simulink model "overhead_crane_linearization_model"  (R2023b)
settings: Solver=VariableStepAuto  StartTime=0.0  StopTime=15  RelTol=1e-3
values from neighbouring files (symbols this model uses):
  A = modello_linearizzazione_Timed_Based_Linearization.a    [linearization_simulink_initialization.m]    (also in overhead_crane_control_initialization.m = overhead_crane_linearization_model_Timed_Based_Linearization)
  alpha_0_eq = pi/2    (= 1.57079632679)    [linearization_simulink_initialization.m]
  alpha_dot_0_eq = 0    [linearization_simulink_initialization.m]
  B = modello_linearizzazione_Timed_Based_Linearization.b    [linearization_simulink_initialization.m]    (also in overhead_crane_control_initialization.m = overhead_crane_linearization_model_Timed_Based_Linearization)
  C = modello_linearizzazione_Timed_Based_Linearization.c    [linearization_simulink_initialization.m]    (also in overhead_crane_control_initialization.m = overhead_crane_linearization_model_Timed_Based_Linearization)
  cc = 5e3    (= 5000)    [linearization_simulink_initialization.m]    (also in overhead_crane_control_initialization.m)
  cm = 100    [linearization_simulink_initialization.m]    (also in overhead_crane_control_initialization.m)
  D = modello_linearizzazione_Timed_Based_Linearization.d    [linearization_simulink_initialization.m]    (also in overhead_crane_control_initialization.m = overhead_crane_linearization_model_Timed_Based_Linearization)
  g = 9.81    [linearization_simulink_initialization.m]    (also in overhead_crane_control_initialization.m)
  L = 2.5    [linearization_simulink_initialization.m]    (also in overhead_crane_control_initialization.m)
  mc = 300    [linearization_simulink_initialization.m]    (also in overhead_crane_control_initialization.m)
  mm = 1000    [linearization_simulink_initialization.m]    (also in overhead_crane_control_initialization.m)
  xc_0_eq = 0    [linearization_simulink_initialization.m]
  xc_dot_0_eq = 0    [linearization_simulink_initialization.m]
undefined symbols (not defined in the file or in its folder): dinamica_alpha
settings Model: Creator=fabio  LastModifiedBy=lorez
settings OptimizationCC: BlockReduction=off  DefaultParameterBehavior=Inlined  BufferReuse=off  ReuseModelBlockBuffer=off

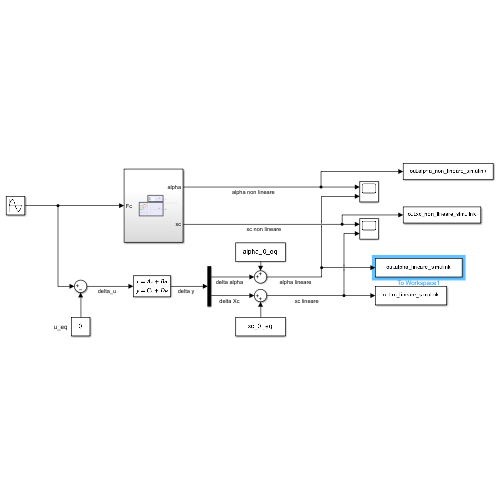
[thumbnail: Simulink's stored preview of the top-level diagram]
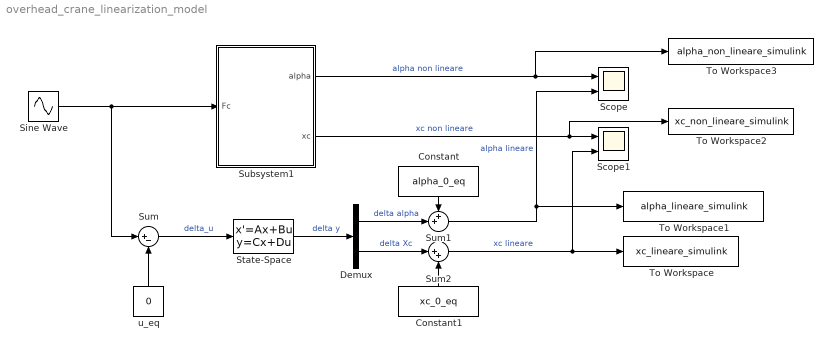
== system overhead_crane_linearization_model ==
  Constant : Constant  Value=alpha_0_eq
  Constant1 : Constant  Value=xc_0_eq
  Demux : Demux  Outputs=2
  Scope : Scope  NumInputPorts=2
  Scope1 : Scope  NumInputPorts=2
  Sine Wave : Sin  Amplitude=1e4  Frequency=2  SampleTime=0
  State-Space : StateSpace  A=A  B=B  C=C  D=D  InitialCondition=0
  Subsystem1 : Subsystem
  Sum : Sum  Inputs=|+-
  Sum1 : Sum  Inputs=++|
  Sum2 : Sum  Inputs=|++
  To Workspace : ToWorkspace  VariableName=xc_lineare_simulink  SampleTime=-1
  To Workspace1 : ToWorkspace  VariableName=alpha_lineare_simulink  SampleTime=-1
  To Workspace2 : ToWorkspace  VariableName=xc_non_lineare_simulink  SampleTime=-1
  To Workspace3 : ToWorkspace  VariableName=alpha_non_lineare_simulink  SampleTime=-1
  u_eq : Constant  Value=0
  wires:
  Subsystem1/1(alpha) -> To Workspace3/1, Scope/1  "alpha non lineare"
  Subsystem1/2(xc) -> To Workspace2/1, Scope1/1  "xc non lineare"
  Sine Wave/1 -> Sum/1, Subsystem1/1(Fc)
  Sum/1 -> State-Space/1  "delta_u"
  u_eq/1 -> Sum/2
  State-Space/1 -> Demux/1  "delta y"
  Demux/1 -> Sum1/2  "delta alpha"
  Constant/1 -> Sum1/1
  Demux/2 -> Sum2/1  "delta Xc"
  Constant1/1 -> Sum2/2
  Sum1/1 -> Scope/2, To Workspace1/1  "alpha lineare"
  Sum2/1 -> Scope1/2, To Workspace/1  "xc lineare"

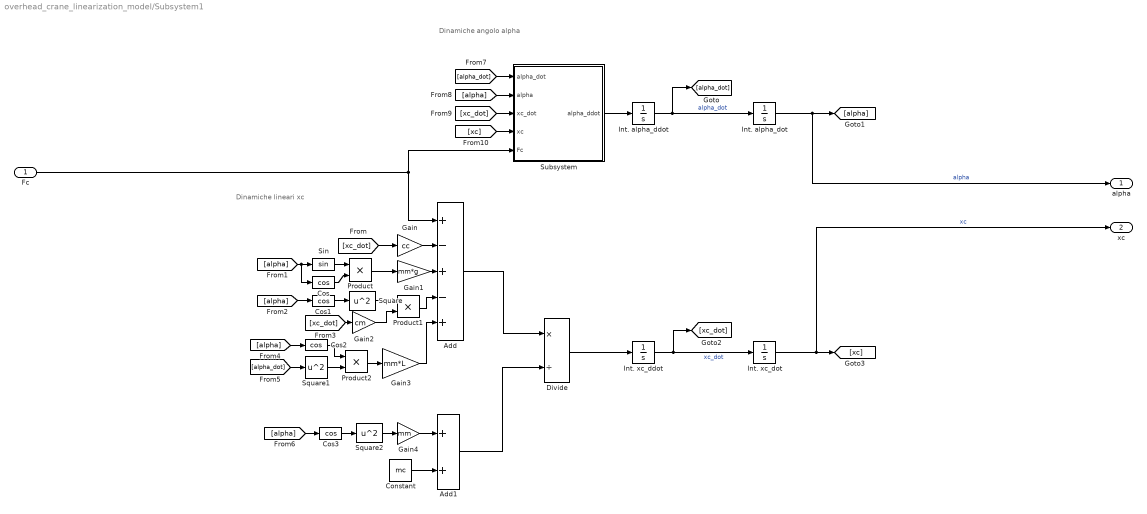
== system overhead_crane_linearization_model/Subsystem1 ==
  note: Dinamiche lineari xc
  note: Dinamiche angolo alpha
  Fc : Inport
  Add : Sum  Inputs=+-+-+
  Add1 : Sum
  Constant : Constant  Value=mc
  Cos{,1..3} (4 alike) : Trigonometry  Operator=cos
  Divide : Product  Inputs=*/
  Gain : Gain  Gain=cc
  Gain1 : Gain  Gain=mm*g
  Gain2 : Gain  Gain=cm
  Gain3 : Gain  Gain=mm*L
  Gain4 : Gain  Gain=mm
  Int. alpha_ddot : Integrator  InitialCondition=alpha_dot_0_eq
  Int. alpha_dot : Integrator  InitialCondition=alpha_0_eq
  Int. xc_ddot : Integrator  InitialCondition=xc_dot_0_eq
  Int. xc_dot : Integrator  InitialCondition=xc_0_eq
  Product : Product
  Product1 : Product
  Product2 : Product
  Sin : Trigonometry
  Square : Math  Operator=square
  Square1 : Math  Operator=square
  Square2 : Math  Operator=square
  Subsystem : Subsystem
  alpha : Outport
  xc : Outport  Port=2
  wires:
  Cos1/1 -> Square/1
  [alpha_dot] -> Subsystem/1(alpha_dot)
  Int. alpha_ddot/1 -> [alpha_dot], Int. alpha_dot/1  "alpha_dot"
  [xc_dot] -> Subsystem/3(xc_dot)
  Square1/1 -> Product2/2
  Int. xc_dot/1 -> xc/1, [xc]  "xc"
  Int. alpha_dot/1 -> alpha/1, [alpha]  "alpha"
  Sin/1 -> Product/1
  Int. xc_ddot/1 -> [xc_dot], Int. xc_dot/1  "xc_dot"
  Fc/1 -> Subsystem/5(Fc), Add/1
  Divide/1 -> Int. xc_ddot/1
  Cos/1 -> Product/2
  Product2/1 -> Gain3/1
  Product/1 -> Gain1/1
  Square/1 -> Product1/1
  [alpha] -> Cos1/1
  [alpha] -> Cos2/1
  [xc_dot] -> Gain/1
  Cos3/1 -> Square2/1
  Product1/1 -> Add/4
  [alpha_dot] -> Square1/1
  Gain2/1 -> Product1/2
  [alpha] -> Subsystem/2(alpha)
  [alpha] -> Cos/1, Sin/1
  Gain1/1 -> Add/3
  [xc_dot] -> Gain2/1
  Add/1 -> Divide/1
  Gain4/1 -> Add1/1
  Gain/1 -> Add/2
  Cos2/1 -> Product2/1
  Add1/1 -> Divide/2
  Gain3/1 -> Add/5
  Subsystem/1(alpha_ddot) -> Int. alpha_ddot/1
  Square2/1 -> Gain4/1
  Constant/1 -> Add1/2
  [xc] -> Subsystem/4(xc)
  [alpha] -> Cos3/1

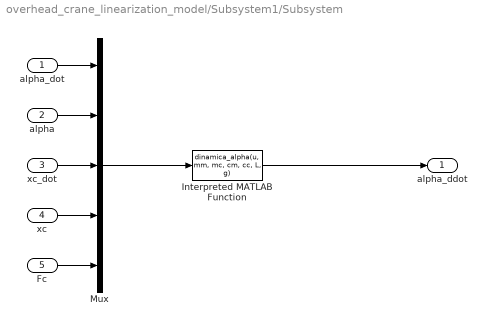
== system overhead_crane_linearization_model/Subsystem1/Subsystem ==
  alpha_dot : Inport
  alpha : Inport  Port=2
  xc_dot : Inport  Port=3
  xc : Inport  Port=4
  Fc : Inport  Port=5
  Interpreted MATLAB Function : MATLABFcn  MATLABFcn=dinamica_alpha(u, mm, mc, cm, cc, L, g)
  Mux : Mux  Inputs=5
  alpha_ddot : Outport
  wires:
  alpha_dot/1 -> Mux/1
  alpha/1 -> Mux/2
  xc_dot/1 -> Mux/3
  xc/1 -> Mux/4
  Fc/1 -> Mux/5
  Mux/1 -> Interpreted MATLAB Function/1
  Interpreted MATLAB Function/1 -> alpha_ddot/1
